simulink model "FCM_test"  (Simulink 7.4)
settings: Solver=FixedStepDiscrete  StartTime=0.0  StopTime=inf  FixedStep=0.01  RelTol=1e-3
undefined symbols (not defined in the file): FCM, FCM_ChaFault_St, FCM_lib, FCMc_i_ConstCurReq, FCMc_i_Currdiff, FCMc_pct_FCMBattType, FCMc_pct_FCMProtolVer, FCMc_pct_PackNominalEnergy, FCMc_pct_PackRatCapacity, FCMc_pct_PackRatVolt, FCMc_pct_PackSocAlwd, FCMc_t_CellTemp_MaxAlwd, FCMc_t_CellTemp_MinAlwd, FCMc_v_CellVolt_MaxAlwd, FCMc_v_CellVolt_MinAlwd, FCMc_v_PackVoltAlwd, FCMc_v_Voltdiff, FCMm_c_CellChaC_AH, FCMm_i_CurrArrayT, FCMx_t_CelltempArrayT
libraries: simulink x13, Defined_Functionality x7
(part 2 of 2)

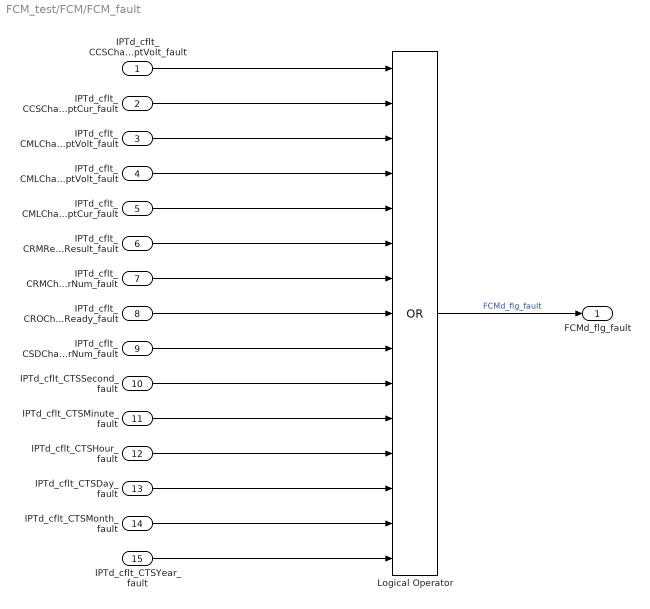
== system FCM_test/FCM/FCM_fault ==
  IPTd_cflt_CCSChagrOptVolt_fault : Inport  OutDataType=fixdt(1, 16)  OutScaling=2^0
  IPTd_cflt_CCSChagrOptCur_fault : Inport  Port=2  OutDataType=fixdt(1, 16)  OutScaling=2^0
  IPTd_cflt_CMLChagrMaxOptVolt_fault : Inport  Port=3  OutDataType=fixdt(1, 16)  OutScaling=2^0
  IPTd_cflt_CMLChagrMinOptVolt_fault : Inport  Port=4  OutDataType=fixdt(1, 16)  OutScaling=2^0
  IPTd_cflt_CMLChagrMaxOptCur_fault : Inport  Port=5  OutDataType=fixdt(1, 16)  OutScaling=2^0
  IPTd_cflt_CRMRecgResult_fault : Inport  Port=6  OutDataType=fixdt(1, 16)  OutScaling=2^0
  IPTd_cflt_CRMChagrSerNum_fault : Inport  Port=7  OutDataType=fixdt(1, 16)  OutScaling=2^0
  IPTd_cflt_CROChagrOptReady_fault : Inport  Port=8  OutDataType=fixdt(1, 16)  OutScaling=2^0
  IPTd_cflt_CSDChagrNum_fault : Inport  Port=9  OutDataType=fixdt(1, 16)  OutScaling=2^0
  IPTd_cflt_CTSSecond_fault : Inport  Port=10  OutDataType=fixdt(1, 16)  OutScaling=2^0
  IPTd_cflt_CTSMinute_fault : Inport  Port=11  OutDataType=fixdt(1, 16)  OutScaling=2^0
  IPTd_cflt_CTSHour_fault : Inport  Port=12  OutDataType=fixdt(1, 16)  OutScaling=2^0
  IPTd_cflt_CTSDay_fault : Inport  Port=13  OutDataType=fixdt(1, 16)  OutScaling=2^0
  IPTd_cflt_CTSMonth_fault : Inport  Port=14  OutDataType=fixdt(1, 16)  OutScaling=2^0
  IPTd_cflt_CTSYear_fault : Inport  Port=15  OutDataType=fixdt(1, 16)  OutScaling=2^0
  Logical Operator : Logic  Operator=OR  Inputs=15  AllPortsSameDT=off  OutDataTypeMode=boolean  LogicDataType=fixdt(0, 8)  OutDataTypeStr=boolean
  FCMd_flg_fault : Outport
  wires:
  IPTd_cflt_CTSYear_fault/1 -> Logical Operator/15
  IPTd_cflt_CTSHour_fault/1 -> Logical Operator/12
  IPTd_cflt_CTSMonth_fault/1 -> Logical Operator/14
  IPTd_cflt_CTSDay_fault/1 -> Logical Operator/13
  IPTd_cflt_CTSMinute_fault/1 -> Logical Operator/11
  IPTd_cflt_CTSSecond_fault/1 -> Logical Operator/10
  IPTd_cflt_CSDChagrNum_fault/1 -> Logical Operator/9
  IPTd_cflt_CROChagrOptReady_fault/1 -> Logical Operator/8
  IPTd_cflt_CRMChagrSerNum_fault/1 -> Logical Operator/7
  IPTd_cflt_CRMRecgResult_fault/1 -> Logical Operator/6
  IPTd_cflt_CMLChagrMaxOptCur_fault/1 -> Logical Operator/5
  IPTd_cflt_CMLChagrMinOptVolt_fault/1 -> Logical Operator/4
  IPTd_cflt_CMLChagrMaxOptVolt_fault/1 -> Logical Operator/3
  IPTd_cflt_CCSChagrOptCur_fault/1 -> Logical Operator/2
  IPTd_cflt_CCSChagrOptVolt_fault/1 -> Logical Operator/1
  Logical Operator/1 -> FCMd_flg_fault/1  "FCMd_flg_fault"

== stateflow chart FCM/FCM_BCL/FCM_BCL ==
  state Timer [function]
    state T1 [function]
      settings: description=$Author:Zhao XiangRi$
      state Run(Limit1) [function]
        settings: description=$Author:Zhao XiangRi$
        (default) -> (junction 16)
        (junction 16) -> (junction 17) [order 1] : [Init1 != 1]
            | {TimeTicks1 = 0;TimeLimit1 = Limit1/10;Init1 = 1;}
        (junction 17) -> (junction 16)
        (junction 16) -> (junction 18) [order 2] : {TimeTicks1++;}
        (junction 18) -> (junction 19) [order 1] : [TimeTicks1 >= TimeLimit1]{Timeout1 = 1;}
        (junction 18) -> (junction 20) [order 2]
      state Clear [function]
        settings: description=$Author:Zhao XiangRi$
        (default) -> (junction 21)
        (junction 21) -> (junction 22) : {Timeout1 = 0;Init1 = 0;}
  state FCM_ConstCurCharging
    state FCM_Init
      en:
      FCMd_flg_ChaStopReq = false;
      FCMd_i_BCLBattChaCurReq = FCMc_i_CurReq_min;
      FCMd_mode_BCLBattChaReq = ConstCurrChaMode;
      FCMd_v_BCLBattChaVoltReq = FCMc_v_PackVoltAlwd;
    state FCM_Curr_Addcout
      du:Timer.T1.Run(FCMc_tm_CurAddDly);
    state FCM_Curr_AddStep
      en:
      FCMd_i_BCLBattChaCurReq +=  FCMc_i_CurReqStep;
      Timer.T1.Clear();
    state FCM_Curr_Const
      en:
      FCMd_i_BCLBattChaCurReq = FCMd_i_ConstCurReq;
    (default) -> FCM_Init
    FCM_Init -> FCM_Curr_Addcout
    (junction 23) -> FCM_Curr_Addcout
    (junction 24) -> (junction 23)
    FCM_Curr_Addcout -> FCM_Curr_AddStep : [Timer.T1.Timeout1 == 1]
    FCM_Curr_AddStep -> (junction 24) [order 2] : [IPTd_i_ShuntCur  <  FCMd_i_ConstCurReq]
    FCM_Curr_AddStep -> FCM_Curr_Const [order 1] : [IPTd_i_ShuntCur  >= FCMd_i_ConstCurReq]
  state FCM_ConstVoltCharging
    state FCM_Curr_Init
      en:
      FCMd_mode_BCLBattChaReq = ConstVoltChaMode;
      FCMd_v_BCLBattChaVoltReq = FCMc_v_PackVoltAlwd ;
      FCMd_i_BCLBattChaCurReq = 0;
    state FCM_CurrExit
      en:
      FCMd_i_BCLBattChaCurReq = FCMc_i_CurReq_min;
      FCMd_flg_ChaStopReq = true;
    (default) -> FCM_Curr_Init
    FCM_Curr_Init -> FCM_CurrExit : [IPTd_i_ShuntCur >= FCMc_i_CurReq_min]
  state FCM_ChaFinished
    en:
    FCMd_flg_ChaStopReq = true;
  (default) -> FCM_ConstCurCharging
  FCM_ConstCurCharging -> FCM_ConstVoltCharging : [(BPNd_v_CellVolt_max >= (FCMc_v_CellVolt_MaxAlwd-FCMc_v_CellVoltDelta))  ...
      | ||(IPTd_v_PosCtrVoltRef1_front >= (FCMc_v_PackVoltAlwd-FCMc_v_PackVoltDelta))]
  FCM_ConstVoltCharging -> FCM_ChaFinished : [(BPNd_v_CellVolt_max >= FCMc_v_CellVolt_MaxAlwd) ...
      |  ||(CORd_pct_PackSoc >= FCMc_pct_PackSocAlwd)]
  data: Timeout1 local boolean; TimeLimit1 local single; TimeTicks1 local single; Init1 local boolean; Limit1 function_input single; FCMc_i_CurReqStep parameter single; FCMc_tm_CurAddDly parameter single; FCMd_i_ConstCurReq input double; IPTd_i_ShuntCur input double; FCMd_v_BCLBattChaVoltReq output int16; FCMd_i_BCLBattChaCurReq output int16; FCMd_mode_BCLBattChaReq output uint8; BPNd_v_CellVolt_max input double; IPTd_v_PosCtrVoltRef1_front input double; CORd_pct_PackSoc input double; FCMc_v_CellVolt_MaxAlwd parameter single; FCMc_v_PackVoltAlwd parameter single; FCMc_pct_PackSocAlwd parameter single; FCMc_v_CellVoltDelta parameter single; FCMc_v_PackVoltDelta parameter single; FCMd_flg_ChaStopReq output boolean; ConstCurrChaMode parameter double; ConstVoltChaMode parameter double; FCMc_i_CurReq_min parameter int16

== stateflow chart FCM/FCM_FLOW ==
  state FCM_Initializating
    en:
    FCMd_enum_ChaSt = FCM_Initializing_St;
    settings: description=$Author:Zhao XiangRi$
  state Timer [function]
    state T1 [function]
      settings: description=$Author:Zhao XiangRi$
      state Run(Limit1) [function]
        settings: description=$Author:Zhao XiangRi$
        (default) -> (junction 98)
        (junction 98) -> (junction 99) [order 1] : [Init1 != 1]
            | {TimeTicks1 = 0;TimeLimit1 = Limit1/10;Init1 = 1;}
        (junction 99) -> (junction 98)
        (junction 98) -> (junction 100) [order 2] : {TimeTicks1++;}
        (junction 100) -> (junction 101) [order 1] : [TimeTicks1 >= TimeLimit1]{Timeout1 = 1;}
        (junction 100) -> (junction 102) [order 2]
      state Clear [function]
        settings: description=$Author:Zhao XiangRi$
        (default) -> (junction 103)
        (junction 103) -> (junction 104) : {Timeout1 = 0;Init1 = 0;}
    state T2 [function]
      settings: description=$Author:Zhao XiangRi$
      state Run(Limit2) [function]
        settings: description=$Author:Zhao XiangRi$
        (default) -> (junction 105)
        (junction 105) -> (junction 106) [order 1] : [Init2 != 1]{TimeTicks2 = 0;TimeLimit2 = Limit2/10 ;Init2 = 1;}
        (junction 106) -> (junction 105)
        (junction 105) -> (junction 107) [order 2] : {TimeTicks2++;}
        (junction 107) -> (junction 108) [order 1] : [TimeTicks2 >= TimeLimit2]{Timeout2 = 1;}
        (junction 107) -> (junction 109) [order 2]
      state Clear [function]
        settings: description=$Author:Zhao XiangRi$
        (default) -> (junction 110)
        (junction 110) -> (junction 111) : {Timeout2 = 0;
            | Init2 = 0;}
  state FCM_HandShaking
    exit:Timer.T1.Clear();Timer.T2.Clear();
    state FCM_HandsShake_Init
      en:
      FCMd_enum_ChaSt = FCM_Handshaking_St;
      du:
      Timer.T1.Run(FCMc_tm_ShakeDly);
    state FCM_HandShake_BEM
      en:
      FCMd_enum_ChaSt = FCM_ChaFault_St;
      FCMd_flg_BEMTM = 1;
    state FCM_HandShake_BRM
      en:
      FCMd_flg_BRMTM = 1;
      du:
      Timer.T2.Run(FCMc_tm_ShakeDly);
    (default) -> FCM_HandsShake_Init
    FCM_HandsShake_Init -> (junction 112) [order 1] : [Timer.T1.Timeout1  == 1 ]%the times to be 5S
    (junction 112) -> FCM_HandShake_BEM : {FCMd_enum_BEMTimeOver3901 = 1;}
    FCM_HandsShake_Init -> (junction 113) [order 2] : [IPTd_flg_CRMRX == true&&Timer.T1.Timeout1 != 1]
    (junction 113) -> (junction 114) [order 2]
    (junction 113) -> FCM_HandShake_BRM [order 1] : [IPTd_enum_CRMRecgResult == 0]
    (junction 114) -> FCM_HandShake_BEM : {FCMd_enum_BEMTimeOver3901 = 2;}
    FCM_HandShake_BRM -> (junction 115) [order 2] : [Timer.T2.Timeout2  == 1]
    (junction 115) -> FCM_HandShake_BEM : {FCMd_enum_BEMTimeOver3902 = 1;}
    (junction 117) -> FCM_HandShake_BEM : {FCMd_enum_BEMTimeOver3902 = 2;}
    FCM_HandShake_BRM -> (junction 116) [order 1] : [IPTd_flg_CRMRX == 1&&...
        | Timer.T2.Timeout2  != 1&&...
        | IPTd_enum_CRMRecgResult != 170]
    (junction 116) -> (junction 117)
  state FCM_ParametesConfiguration
    exit:Timer.T2.Clear();Timer.T1.Clear();
    state FCM_Config_BCP
      en:
      FCMd_enum_ChaSt = FCM_Configuration_St;
      FCMd_flg_BCPTM = 1;
      du:
      Timer.T1.Run(FCMc_tm_ConfigDly);
    state FCM_Config_BROExit
      en:
      FCMd_flg_BROTM = 1;
      FCMd_enum_BROBattChaReady = 0;
      FCMd_enum_ChaSt = FCM_ChaFault_St;
    state FCM_Config_BROIn
      en:
      FCMd_enum_BROBattChaReady = 170;
      FCMd_flg_BROTM = 1;
      du:
      Timer.T2.Run(FCMc_tm_ConfigDly);
    state FCM_Config_BEM
      en:
      FCMd_flg_BEMTM = 1;
      FCMd_enum_ChaSt = FCM_ChaFault_St;
    state FCM_Config_Exit
      du:
      FCMd_enum_ChaCtrCmd = CTC_FastChaOnline_CtrCmd;
    FCM_Config_BCP -> (junction 118) [order 2] : [Timer.T1.Timeout1  == 1]
    (junction 118) -> FCM_Config_BEM : {FCMd_enum_BEMTimeOver3903 = 1;}
    FCM_Config_BCP -> (junction 119) [order 1] : [IPTd_flg_CTSRX == 1 ...
        |  && IPTd_flg_CMLRX == 1 ...
        |  && Timer.T1.Timeout1  != 1]%need cts and cms both receive
    (junction 121) -> FCM_Config_BEM : {FCMd_enum_BEMTimeOver3903 = 2;}
    (junction 122) -> FCM_Config_BEM : {FCMd_enum_BEMTimeOver3904 = 1;}
    (junction 123) -> FCM_Config_BEM : {FCMd_enum_BEMTimeOver3904 = 2;}
    (junction 119) -> FCM_Config_BROExit [order 2] : [FCMd_flg_BSMChaAlwd == 0]
    (junction 119) -> (junction 120) [order 1] : [FCMd_flg_BSMChaAlwd == 1]
    (junction 120) -> (junction 121) [order 2]
    (junction 120) -> FCM_Config_BROIn [order 1] : [FCMd_cflt_CTS == 0 ...
        |  && FCMd_cflt_CML == 0]%need charge enable
    FCM_Config_BROIn -> (junction 122) [order 2] : [ Timer.T2.Timeout2  == 1]%the times  to be 5S
    (junction 124) -> FCM_Config_BROIn
    FCM_Config_BROIn -> (junction 125) [order 1] : [IPTd_flg_CRORX == 1 ...
        |  && Timer.T2.Timeout2  != 1]
    (junction 125) -> (junction 123) [order 2] : [FCMd_cflt_CRO == 1]
    (junction 125) -> (junction 124) [order 3] : [IPTd_enum_CROChagrOptReady == 0 ...
        |  || IPTd_enum_CROChagrOptReady == 255]
    (junction 125) -> FCM_Config_Exit [order 1] : [IPTd_enum_CROChagrOptReady == 170]
    (default) -> FCM_Config_BCP
  state FCM_Charging
    exit:Timer.T1.Clear();
    state FCM_Charging_BCL
      en:
      FCMd_enum_ChaSt = FCM_Charging_St;
      FCMd_flg_BCLTM  = 1;
      FCMd_flg_BCSTM = 1;
      du:
      Timer.T1.Run(FCMc_tm_ChaDly);
    state FCM_Charging_BEM
      en:
      FCMd_enum_ChaSt = FCM_ChaFault_St ;
      FCMd_flg_BEMTM = 1;
    state FCM_Charging_BSM
      en:
      FCMd_flg_BSMTM = 1;
      FCMd_flg_BMVTM = 1;
      FCMd_flg_BMTTM = 1;
      Timer.T1.Clear();
    (junction 126) -> FCM_Charging_BCL
    FCM_Charging_BCL -> (junction 127) [order 2] : [Timer.T1.Timeout1  == 1]%the times  to be 100ms
    (junction 130) -> (junction 126)
    (junction 127) -> FCM_Charging_BEM : {FCMd_enum_BEMTimeOver3905 = 1;}
    FCM_Charging_BCL -> (junction 128) [order 1] : [IPTd_flg_CCSRX == 1 ...
        | && Timer.T1.Timeout1  != 1]
    (junction 128) -> (junction 129) [order 1] : [FCMd_cflt_CCS == 1]
    (junction 128) -> FCM_Charging_BSM [order 2] : [FCMd_cflt_CCS == 0]
    (junction 129) -> FCM_Charging_BEM : {FCMd_enum_BEMTimeOver3905 = 2;}
    FCM_Charging_BSM -> (junction 131)
    (junction 131) -> (junction 130) : [FCMd_flg_BSMChaAlwd == 1 ...
        | && IPTd_flg_CSTRX == 0]
    (default) -> FCM_Charging_BCL
  state FCM_Finished
    exit:Timer.T1.Clear();Timer.T2.Clear();
    state FCM_Finished_Init
      en:
      FCMd_enum_ChaSt =FCM_ChaFinished_St;
      FCMd_flg_BSTTM = 1;
      du:Timer.T1.Run(FCMc_tm_FinishDly);
    state FCM_Finished_BEM
      en:
      FCMd_flg_BEMTM = 1;
      FCMd_enum_ChaSt = FCM_ChaFault_St;
      FCMd_enum_ChaCtrCmd = CTC_FastChaOffline_CtrCmd;
    state FCM_Finished_Exit
      en:
      FCMd_enum_ChaCtrCmd = CTC_FastChaOffline_CtrCmd;
    state FCM_Finished_BSD
      en:
      FCMd_flg_BSDTM = 1;
      du:Timer.T2.Run(FCMc_tm_FinishDly);
    (default) -> FCM_Finished_Init
    FCM_Finished_Init -> (junction 132) [order 2] : [Timer.T1.Timeout1  == 1]
    (junction 132) -> FCM_Finished_BEM : {FCMd_enum_BEMTimeOver3906 = 1;}
    FCM_Finished_Init -> (junction 133) [order 1] : [IPTd_flg_CSTRX == 1 ...
        |  && Timer.T1.Timeout1  != 1 ]
    (junction 133) -> (junction 134) [order 2]
    (junction 133) -> FCM_Finished_BSD [order 1] : [FCMd_cflt_CST == 0]
    (junction 134) -> FCM_Finished_BEM : {FCMd_enum_BEMTimeOver3906 = 2;}
    FCM_Finished_BSD -> (junction 135) [order 2] : [Timer.T2.Timeout2 == 1]
    (junction 135) -> FCM_Finished_BEM : {FCMd_enum_BEMTimeOver3907 = 1;}
    FCM_Finished_BSD -> (junction 136) [order 1] : [IPTd_flg_CSDRX == 1 ...
        | &&Timer.T2.Timeout2 != 1]
    (junction 136) -> (junction 137) [order 2]
    (junction 136) -> FCM_Finished_Exit [order 1] : [FCMd_cflt_CSD == 0]
    (junction 137) -> FCM_Finished_BEM : {FCMd_enum_BEMTimeOver3907 = 2;}
  (junction 143) -> FCM_Finished
  FCM_Finished -> (junction 144) : [CTCd_enum_CtrSt==CTC_FastChaOffline_St...
      | &&FCMd_enum_ChaCtrCmd == CTC_FastChaOffline_CtrCmd]
  FCM_HandShaking -> FCM_ParametesConfiguration [order 2] : [IPTd_flg_CRMRX == 1&&...
      | IPTd_enum_CRMRecgResult== 170]
  (junction 142) -> (junction 143)
  (default) -> FCM_Initializating
  (junction 141) -> (junction 140)
  (junction 144) -> (junction 138)
  (junction 139) -> FCM_Initializating
  (junction 140) -> (junction 139)
  FCM_Initializating -> FCM_HandShaking : [BSCd_enum_BCUSt==BCU_FastCharge_St]
  FCM_HandShaking -> (junction 140) [order 1] : [FCMd_enum_ChaSt == FCM_ChaFault_St]
  FCM_ParametesConfiguration -> (junction 141) [order 1] : [FCMd_enum_ChaSt == FCM_ChaFault_St]
  FCM_Charging -> FCM_Finished [order 2] : [FCMd_flg_BSMChaAlwd == 0 ...
      | && IPTd_flg_CSTRX == 1]
  FCM_ParametesConfiguration -> FCM_Charging [order 2] : [CTCd_enum_CtrSt==CTC_FastChaOnline_St ...
      | &&FCMd_enum_ChaCtrCmd == CTC_FastChaOnline_CtrCmd]
  FCM_Charging -> (junction 142) [order 1] : [FCMd_enum_ChaSt == FCM_ChaFault_St]
  (junction 138) -> (junction 139)
  data: Timeout1 local boolean; TimeLimit1 local single; Init1 local boolean; TimeTicks1 local single; Limit1 function_input single; Timeout2 local boolean; TimeLimit2 local single; TimeTicks2 local single; Init2 local boolean; Limit2 function_input single; BCU_FastCharge_St parameter uint8; CTC_FastChaOffline_CtrCmd parameter uint8; CTC_FastChaOnline_CtrCmd parameter uint8; CTC_FastChaOnline_St parameter uint8; CTC_FastChaOffline_St parameter uint8; BSCd_enum_BCUSt input uint8; IPTd_enum_CRMRecgResult input double; IPTd_enum_CROChagrOptReady input double; CTCd_enum_CtrSt input uint8; FCMd_flg_BSMChaAlwd input boolean; FCM_Initializing_St parameter uint8; FCM_Handshaking_St parameter uint8; FCM_Configuration_St parameter uint8; FCM_Charging_St parameter uint8; FCM_ChaFinished_St parameter uint8; FCM_ChaFault_St parameter uint8; IPTd_flg_CCSRX input boolean; IPTd_flg_CMLRX input boolean; IPTd_flg_CRORX input boolean; IPTd_flg_CSDRX input boolean; IPTd_flg_CSTRX input boolean; IPTd_flg_CTSRX input boolean; IPTd_flg_CRMRX input boolean; FCMd_enum_BEMTimeOver3901 output uint8; FCMd_enum_BEMTimeOver3902 output uint8; FCMd_enum_BEMTimeOver3903 output uint8; FCMd_enum_BEMTimeOver3904 output uint8; FCMd_enum_BEMTimeOver3905 output uint8; FCMd_enum_BEMTimeOver3906 output uint8; FCMd_enum_BEMTimeOver3907 output uint8; FCMd_flg_BRMTM output boolean; FCMd_flg_BCPTM output boolean; FCMd_flg_BROTM output boolean; FCMd_flg_BCLTM output boolean; FCMd_flg_BCSTM output boolean; FCMd_flg_BSMTM output boolean; FCMd_flg_BMVTM output boolean; FCMd_flg_BMTTM output boolean; FCMd_flg_BSTTM output boolean; FCMd_flg_BSDTM output boolean; FCMd_flg_BEMTM output boolean; FCMd_enum_ChaCtrCmd output uint8; FCMd_enum_BROBattChaReady output uint8; FCMd_enum_ChaSt output uint8; FCMc_tm_ShakeDly parameter uint16; FCMc_tm_ConfigDly parameter uint16; FCMc_tm_ChaDly parameter uint16; FCMc_tm_FinishDly parameter uint16; FCMd_cflt_CCS input double; FCMd_cflt_CML input double; FCMd_cflt_CRO input double; FCMd_cflt_CSD input double; FCMd_cflt_CST input double; FCMd_cflt_CTS input double
